simulink model "Control_Vehiculo_new_MCI_MCD"  (R2022a)
settings: Solver=FixedStepAuto  StartTime=0.0  StopTime=inf  MaxStep=0.01  RelTol=1e-3  EnableMultiTasking=on
InitFcn:
  | R=0.0875;
  | Lx=0.24;
  | Ly=0.279;
  | b=0.558;
  | r=R;
  | Ts=0.01;
  | cal_time=1;
libraries: simulink x6, simulink_need_slupdate x1, slpidlib x1, arduinolib x1
settings Model: ExtModeTrigDuration=2  Creator=eva_g  LastModifiedBy=Nuc1
settings SolverCC: AlgebraicLoopSolver=TrustRegion
settings OptimizationCC: EnhancedBackFolding=on  PassReuseOutputArgsAs=Individual arguments  ZeroExternalMemoryAtStartup=off  ZeroInternalMemoryAtStartup=off  MaxStackSize=64  OptimizeBlockOrder=speed  DifferentSizesBufferReuse=on  OptimizationCustomize=off  EfficientTunableParamExpr=on
settings DebuggingCC: ParameterTunabilityLossMsg=error  UnconnectedInputMsg=warning  UnconnectedOutputMsg=warning  UnconnectedLineMsg=warning  SFMachineParentedDataDiag=warning
settings HardwareCC: ProdBitPerInt=16  ProdBitPerPointer=16  ProdBitPerSizeT=16  ProdBitPerPtrDiffT=16  ProdLargestAtomicFloat=None  ProdWordSize=8  ProdHWDeviceType=Atmel->AVR
settings SFSimCC: MATLABDynamicMemAlloc=off
settings RTWCC: SystemTargetFile=ert.tlc  HardwareBoard=Arduino Mega 2560  TemplateMakefile=ert_default_tmf  Toolchain=Arduino AVR  BuildConfiguration=Faster Runs  DLArmComputeVersion=19.05
settings CodeAppCC: ForceParamTrailComments=on  IgnoreCustomStorageClasses=off  OperatorAnnotations=on  SimulinkDataObjDesc=on  SFDataObjDesc=on  InsertBlockDesc=on
settings ERTTargetCC: SupportContinuousTime=on  SupportVariableSizeSignals=on  ExtModeStaticAllocSize=2048

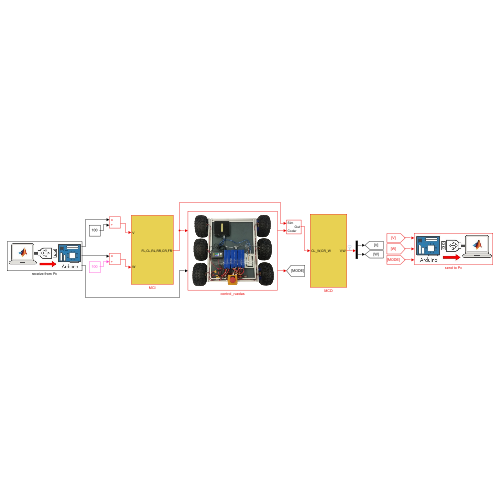
[thumbnail: Simulink's stored preview of the top-level diagram]
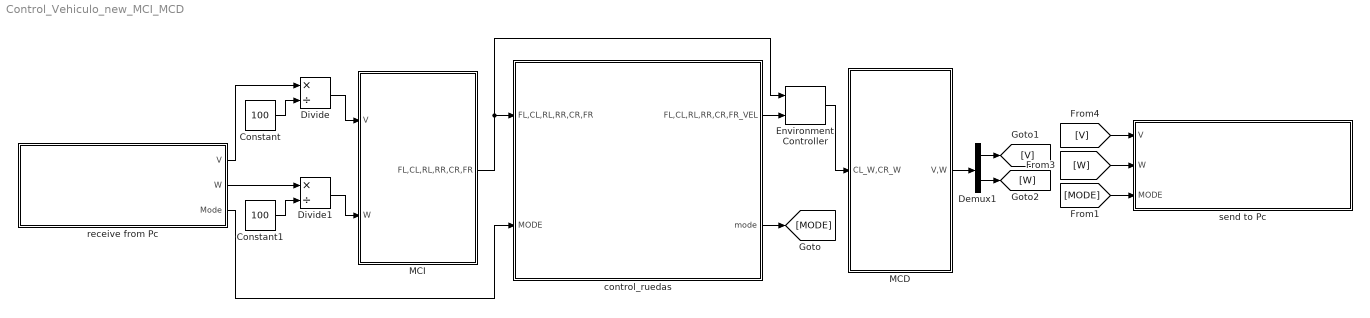
== system Control_Vehiculo_new_MCI_MCD ==
  Constant : Constant  Value=100  OutDataTypeStr=single
  Constant1 : Constant  Value=100  OutDataTypeStr=single
  Demux1 : Demux  Outputs=2
  Divide : Product  Inputs=*/
  Divide1 : Product  Inputs=*/
  Environment Controller : simulink_need_slupdate/Environment Controller
      settings: SourceProductBaseCode=SL
  MCD : Subsystem
  MCI : Subsystem
  control_ruedas : Subsystem
      mask Display: image('ruedas1.png'); % Use "Edit Image" on toolstrip to change.
  receive from Pc : Subsystem
      mask Display: image('ma.jpg'); % Use "Edit Image" on toolstrip to change.
  send to Pc : Subsystem
      mask Display: image('am.jpg'); % Use "Edit Image" on toolstrip to change.
  wires:
  [V] -> send to Pc/1(V)
  Divide1/1 -> MCI/2(W)
  Constant/1 -> Divide/2
  Divide/1 -> MCI/1(V)
  control_ruedas/1(FL,CL,RL,RR,CR,FR_VEL) -> Environment Controller/2
  MCI/1(FL,CL,RL,RR,CR,FR) -> control_ruedas/1(FL,CL,RL,RR,CR,FR), Environment Controller/1
  Environment Controller/1 -> MCD/1(CL_W,CR_W)
  Constant1/1 -> Divide1/2
  control_ruedas/2(mode) -> [MODE]
  Demux1/2 -> [W]
  [MODE] -> send to Pc/3(MODE)
  Demux1/1 -> [V]
  [W] -> send to Pc/2(W)
  MCD/1(V,W) -> Demux1/1
  receive from Pc/1(V) -> Divide/1
  receive from Pc/2(W) -> Divide1/1
  receive from Pc/3(Mode) -> control_ruedas/2(MODE)

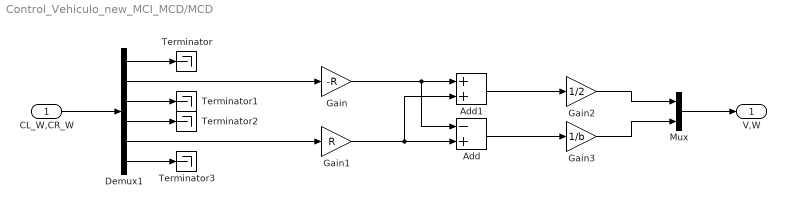
== system Control_Vehiculo_new_MCI_MCD/MCD ==
  CL_W,CR_W : Inport
  Add : Sum  Inputs=-+
  Add1 : Sum
  Demux1 : Demux  Outputs=6
  Gain : Gain  Gain=-R
  Gain1 : Gain  Gain=R
  Gain2 : Gain  Gain=1/2
  Gain3 : Gain  Gain=1/b  ParamDataTypeStr=double
  Mux : Mux  Inputs=2
  Terminator{,1..3} (4 alike) : Terminator
  V,W : Outport
  wires:
  Gain1/1 -> Add/2, Add1/2
  Gain/1 -> Add/1, Add1/1
  Add/1 -> Gain3/1
  Add1/1 -> Gain2/1
  Gain2/1 -> Mux/1
  Gain3/1 -> Mux/2
  Mux/1 -> V,W/1
  CL_W,CR_W/1 -> Demux1/1
  Demux1/2 -> Gain/1
  Demux1/5 -> Gain1/1
  Demux1/1 -> Terminator/1
  Demux1/3 -> Terminator1/1
  Demux1/4 -> Terminator2/1
  Demux1/6 -> Terminator3/1

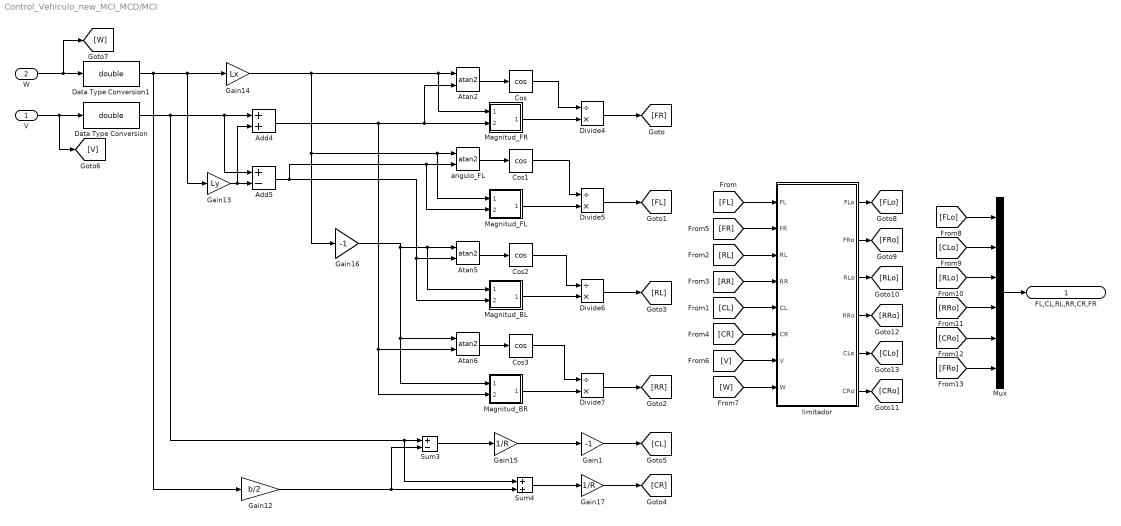
== system Control_Vehiculo_new_MCI_MCD/MCI ==
  V : Inport
  W : Inport  Port=2
  Add4 : Sum
  Add5 : Sum  Inputs=+-
  Atan2 : Trigonometry  Operator=atan2
  Atan5 : Trigonometry  Operator=atan2
  Atan6 : Trigonometry  Operator=atan2
  Cos{,1..3} (4 alike) : Trigonometry  Operator=cos
  Data Type Conversion : DataTypeConversion  OutDataTypeStr=double  SaturateOnIntegerOverflow=off  RndMeth=Floor
  Data Type Conversion1 : DataTypeConversion  OutDataTypeStr=double  SaturateOnIntegerOverflow=off  RndMeth=Floor
  Divide{4..7} (4 alike) : Product  Inputs=/*
  Gain1 : Gain  Gain=-1
  Gain12 : Gain  Gain=b/2
  Gain13 : Gain  Gain=Ly
  Gain14 : Gain  Gain=Lx
  Gain15 : Gain  Gain=1/R
  Gain16 : Gain  Gain=-1
  Gain17 : Gain  Gain=1/R
  Magnitud_BL : Subsystem
  Magnitud_BR : Subsystem
  Magnitud_FL : Subsystem
  Magnitud_FR : Subsystem
  Mux : Mux  Inputs=6
  Sum3 : Sum  Inputs=+-
  Sum4 : Sum
  angulo_FL : Trigonometry  Operator=atan2
  limitador : MATLAB Function  TreatAsAtomicUnit=on
  FL,CL,RL,RR,CR,FR : Outport
  wires:
  Cos/1 -> Divide4/1
  Sum3/1 -> Gain15/1
  Cos3/1 -> Divide7/1
  Sum4/1 -> Gain17/1
  W/1 -> [W], Data Type Conversion1/1
  Gain14/1 -> Magnitud_FR/1(In1), Atan2/1, angulo_FL/1, Magnitud_FL/1(In1), Gain16/1
  Magnitud_FL/1(w_FL) -> Divide5/2
  Atan5/1 -> Cos2/1
  Gain12/1 -> Sum4/2, Sum3/2
  Gain16/1 -> Atan5/1, Magnitud_BL/1(In1), Atan6/1, Magnitud_BR/1(In1)
  Add5/1 -> angulo_FL/2, Magnitud_FL/2(In2), Atan5/2, Magnitud_BL/2(In2)
  Gain15/1 -> Gain1/1
  Add4/1 -> Atan6/2, Magnitud_BR/2(In2), Atan2/2, Magnitud_FR/2(In2)
  angulo_FL/1 -> Cos1/1
  Magnitud_BL/1(w_BL) -> Divide6/2
  Gain13/1 -> Add4/2, Add5/2
  V/1 -> [V], Data Type Conversion/1
  Cos2/1 -> Divide6/1
  Cos1/1 -> Divide5/1
  Magnitud_BR/1(w_BR) -> Divide7/2
  Magnitud_FR/1(w_FR) -> Divide4/2
  Atan6/1 -> Cos3/1
  Atan2/1 -> Cos/1
  Mux/1 -> FL,CL,RL,RR,CR,FR/1
  Divide4/1 -> [FR]
  Divide5/1 -> [FL]
  Divide6/1 -> [RL]
  Gain1/1 -> [CL]
  Gain17/1 -> [CR]
  Data Type Conversion/1 -> Sum4/1, Sum3/1, Add5/1, Add4/1
  Data Type Conversion1/1 -> Gain12/1, Gain14/1, Gain13/1
  Divide7/1 -> [RR]
  [CR] -> limitador/6(CR)
  [FR] -> limitador/2(FR)
  [CL] -> limitador/5(CL)
  [RL] -> limitador/3(RL)
  [FL] -> limitador/1(FL)
  [RR] -> limitador/4(RR)
  [V] -> limitador/7(V)
  [W] -> limitador/8(W)
  limitador/1(FLo) -> [FLo]
  limitador/2(FRo) -> [FRo]
  limitador/3(RLo) -> [RLo]
  limitador/4(RRo) -> [RRo]
  limitador/5(CLo) -> [CLo]
  limitador/6(CRo) -> [CRo]
  [FLo] -> Mux/1
  [CLo] -> Mux/2
  [RLo] -> Mux/3
  [CRo] -> Mux/5
  [FRo] -> Mux/6
  [RRo] -> Mux/4

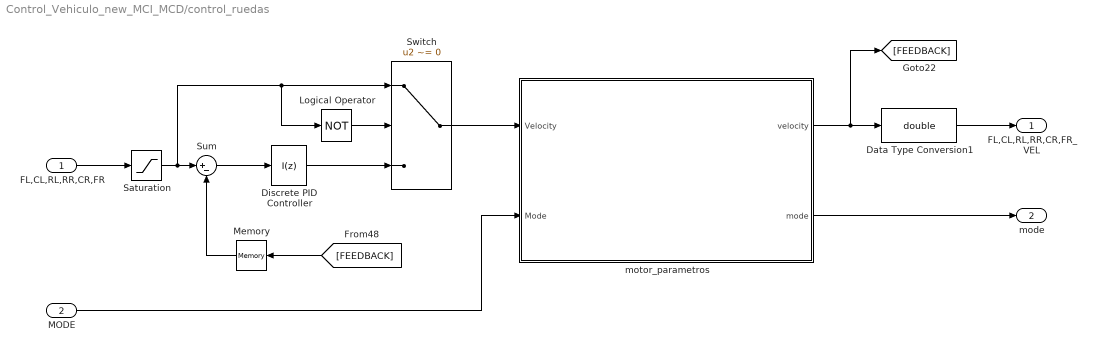
== system Control_Vehiculo_new_MCI_MCD/control_ruedas ==
  FL,CL,RL,RR,CR,FR : Inport
  MODE : Inport  Port=2
  Data Type Conversion1 : DataTypeConversion  OutDataTypeStr=double  SaturateOnIntegerOverflow=off  RndMeth=Floor
  Discrete PID Controller : slpidlib/PID Controller  Controller=I  Form=Parallel  TimeDomain=Discrete-time  UseExternalTs=off  SampleTime=-1  IntegratorMethod=Forward Euler  FilterMethod=Forward Euler  ControllerParametersSource=internal  P=0.7  I=10  UseKiTs=off  D=0  N=100  UseFilter=on  TunerSelectOption=Transfer Function Based (PID Tuner App)  InitialConditionSource=internal  InitialConditionForIntegrator=0  InitialConditionForFilter=0  DifferentiatorICPrevScaledInput=0  ExternalReset=none  TrackingMode=off  Kt=1  LimitOutput=on  SatLimitsSource=internal  UpperSaturationLimit=10  LowerSaturationLimit=-10  LinearizeAsGain=on  AntiWindupMode=clamping  Kb=1  POutMin=[]  POutMax=[]  IOutMin=[]  IOutMax=[]  DOutMin=[]  DOutMax=[]  NOutMin=[]  NOutMax=[]  SumOutMin=[]  SumOutMax=[]  SaturationOutMin=[]  SaturationOutMax=[]  PParamMin=[]  PParamMax=[]  IParamMin=[]  IParamMax=[]  DParamMin=[]  DParamMax=[]  NParamMin=[]  NParamMax=[]  KbParamMin=[]  KbParamMax=[]  KtParamMin=[]  KtParamMax=[]  KbOutMin=[]  KbOutMax=[]  KtOutMin=[]  KtOutMax=[]  IntegratorOutMin=[]  IntegratorOutMax=[]  FilterOutMin=[]  FilterOutMax=[]  SumI1OutMin=[]  SumI1OutMax=[]  SumI2OutMin=[]  SumI2OutMax=[]  SumI3OutMin=[]  SumI3OutMax=[]  SumI4OutMin=[]  SumI4OutMax=[]  SumDOutMin=[]  SumDOutMax=[]  DifferentiatorOutMin=[]  DifferentiatorOutMax=[]  FilterDiffOutCoefMin=[]  FilterDiffOutCoefMax=[]  ReciprocalOutMin=[]  ReciprocalOutMax=[]  SumDenOutMin=[]  SumDenOutMax=[]  SumNumOutMin=[]  SumNumOutMax=[]  DivideOutMin=[]  DivideOutMax=[]  UdiffTsProdOutMin=[]  UdiffTsProdOutMax=[]  NTsProdOutMin=[]  NTsProdOutMax=[]  UintegralTsProdOutMin=[]  UintegralTsProdOutMax=[]  UngainTsProdOutMin=[]  UngainTsProdOutMax=[]  IntegratorContinuousStateAttributes=''  IntegratorStateMustResolveToSignalObject=off  IntegratorRTWStateStorageClass=Auto  FilterContinuousStateAttributes=''  FilterStateMustResolveToSignalObject=off  FilterRTWStateStorageClass=Auto  ParallelPVariant=Disabled  IdealPVariant=Disabled  IVariant=InternalParameters  DVariant=Disabled  IntegratorVariant=Discrete  SatVariant=Enabled  AWVariant=DiscClampingParallel  PCopyVariant=Disabled  TRVariant=Disabled  FdbkBlocksVariant=Forward  IdealPFdbkVariant=Disabled  SatFdbkVariant=Disabled  DerivativeFilterVariant=Disabled  NVariant=Disabled  NCopyVariant=Disabled_SignalSpec  FilterICVariant=Disabled  IntegratorICVariant=InternalICs  ExternalResetVariant=Disabled  TRSumVariant=Passthrough  SumFdbkVariant=Disabled  SumVariant=Passthrough_I  TsampFilterVariant=InternalTs  TsampNgainVariant=Passthrough  TsampIntegralVariant=Passthrough  ExternalSaturationOutDataTypeStr=Inherit: Same as second input  aMode=0
  Logical Operator : Logic  Operator=NOT  AllPortsSameDT=off  OutDataTypeStr=boolean
  Memory : Memory
  Saturation : Saturate  UpperLimit=10  LowerLimit=-10
  Sum : Sum  Inputs=|+-
  Switch : Switch  Criteria=u2 ~= 0  SaturateOnIntegerOverflow=off  InputSameDT=off
  motor_parametros : Subsystem
  FL,CL,RL,RR,CR,FR_VEL : Outport
  mode : Outport  Port=2
  wires:
  Memory/1 -> Sum/2
  Sum/1 -> Discrete PID Controller/1
  Discrete PID Controller/1 -> Switch/3
  [FEEDBACK] -> Memory/1
  Data Type Conversion1/1 -> FL,CL,RL,RR,CR,FR_VEL/1
  Logical Operator/1 -> Switch/2
  FL,CL,RL,RR,CR,FR/1 -> Saturation/1
  Saturation/1 -> Logical Operator/1, Switch/1, Sum/1
  motor_parametros/1(velocity) -> [FEEDBACK], Data Type Conversion1/1
  MODE/1 -> motor_parametros/2(Mode)
  motor_parametros/2(mode) -> mode/1
  Switch/1 -> motor_parametros/1(Velocity)

== system Control_Vehiculo_new_MCI_MCD/receive from Pc ==
  receive from Pc : S-Function  InitFcn=try, set_param(gcb,'FunctionName','receive_serial'), end  FunctionName=receive_serial  SFunctionModules=receive_serial_wrapper  SFunctionDeploymentMode=off  EnableBusSupport=off  mask(S-Function Builder){}
      mask help: Simulink:masks:SFunctionBuilder_MD
      mask init:
      | val = [[.9  0.75 0.75 1 1 .9 .9 1]',[1 1 0.75 0.75 .9 .9 1 .9]'];try , sys = get_param(gcb,'SfunBuilderFcnName');if isempty(sys), sys = get_param(gcb,'FunctionName'); end,catch, sys = get_param(gcb,'FunctionName'); end
      settings: CopyFcn=set_param(gcbh,'LinkStatus','none')  PreSaveFcn=try, set_param(gcb,'FunctionName','receive_serial'), end  OpenFcn=sfunctionwizard(gcbh)
      mask Display: plot(val(:,1),val(:,2)),disp(sys),port_label('output',1,'v'),port_label('output',2,'w'),port_label('output',3,'m')
  V : Outport
  W : Outport  Port=2
  Mode : Outport  Port=3
  wires:
  receive from Pc/2 -> W/1
  receive from Pc/1 -> V/1
  receive from Pc/3 -> Mode/1

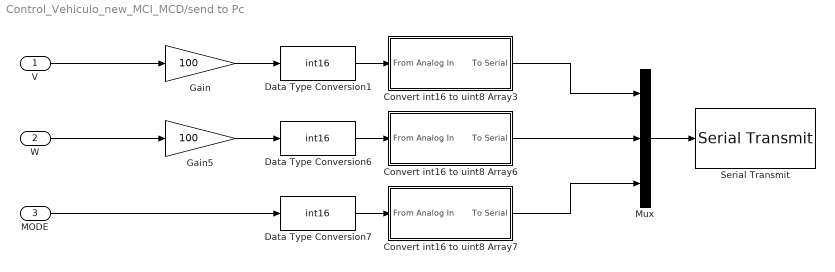
== system Control_Vehiculo_new_MCI_MCD/send to Pc ==
  V : Inport
  W : Inport  Port=2
  MODE : Inport  Port=3
  Convert int16 to uint8 Array3 : Subsystem
  Convert int16 to uint8 Array6 : Subsystem
  Convert int16 to uint8 Array7 : Subsystem
  Data Type Conversion1 : DataTypeConversion  OutDataTypeStr=int16  ConvertRealWorld=Stored Integer (SI)  SaturateOnIntegerOverflow=off  RndMeth=Floor
  Data Type Conversion6 : DataTypeConversion  OutDataTypeStr=int16  ConvertRealWorld=Stored Integer (SI)  SaturateOnIntegerOverflow=off  RndMeth=Floor
  Data Type Conversion7 : DataTypeConversion  OutDataTypeStr=int16  ConvertRealWorld=Stored Integer (SI)  SaturateOnIntegerOverflow=off  RndMeth=Floor
  Gain : Gain  Gain=100
  Gain5 : Gain  Gain=100
  Mux : Mux  Inputs=3
  Serial Transmit : arduinolib/Serial Transmit  portNumber=0  sendmode=write  sendformat=Decimal  floatprecision=2  blockPlatform=arduino
  wires:
  Convert int16 to uint8 Array7/1(To Serial) -> Mux/3
  Data Type Conversion7/1 -> Convert int16 to uint8 Array7/1(From Analog In)
  MODE/1 -> Data Type Conversion7/1
  W/1 -> Gain5/1
  V/1 -> Gain/1
  Convert int16 to uint8 Array3/1(To Serial) -> Mux/1
  Convert int16 to uint8 Array6/1(To Serial) -> Mux/2
  Gain5/1 -> Data Type Conversion6/1
  Data Type Conversion6/1 -> Convert int16 to uint8 Array6/1(From Analog In)
  Gain/1 -> Data Type Conversion1/1
  Data Type Conversion1/1 -> Convert int16 to uint8 Array3/1(From Analog In)
  Mux/1 -> Serial Transmit/1

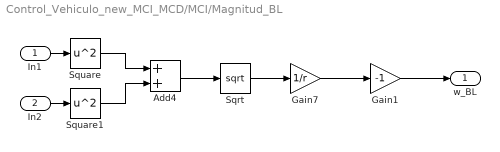
== system Control_Vehiculo_new_MCI_MCD/MCI/Magnitud_BL ==
  In1 : Inport
  In2 : Inport  Port=2
  Add4 : Sum
  Gain1 : Gain  Gain=-1
  Gain7 : Gain  Gain=1/r
  Sqrt : Sqrt
  Square : Math  Operator=square
  Square1 : Math  Operator=square
  w_BL : Outport
  wires:
  Sqrt/1 -> Gain7/1
  Square1/1 -> Add4/2
  In2/1 -> Square1/1
  Add4/1 -> Sqrt/1
  Square/1 -> Add4/1
  In1/1 -> Square/1
  Gain7/1 -> Gain1/1
  Gain1/1 -> w_BL/1

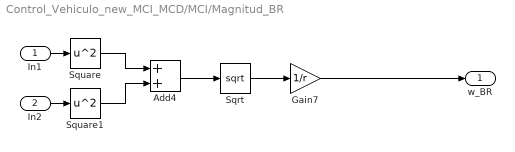
== system Control_Vehiculo_new_MCI_MCD/MCI/Magnitud_BR ==
  In1 : Inport
  In2 : Inport  Port=2
  Add4 : Sum
  Gain7 : Gain  Gain=1/r
  Sqrt : Sqrt
  Square : Math  Operator=square
  Square1 : Math  Operator=square
  w_BR : Outport
  wires:
  In1/1 -> Square/1
  Square/1 -> Add4/1
  Add4/1 -> Sqrt/1
  In2/1 -> Square1/1
  Square1/1 -> Add4/2
  Sqrt/1 -> Gain7/1
  Gain7/1 -> w_BR/1

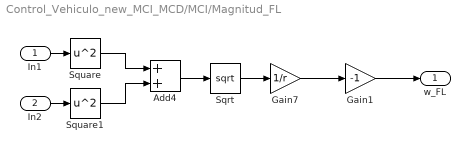
== system Control_Vehiculo_new_MCI_MCD/MCI/Magnitud_FL ==
  In1 : Inport
  In2 : Inport  Port=2
  Add4 : Sum
  Gain1 : Gain  Gain=-1
  Gain7 : Gain  Gain=1/r
  Sqrt : Sqrt
  Square : Math  Operator=square
  Square1 : Math  Operator=square
  w_FL : Outport
  wires:
  Square1/1 -> Add4/2
  In2/1 -> Square1/1
  Add4/1 -> Sqrt/1
  Square/1 -> Add4/1
  In1/1 -> Square/1
  Sqrt/1 -> Gain7/1
  Gain7/1 -> Gain1/1
  Gain1/1 -> w_FL/1

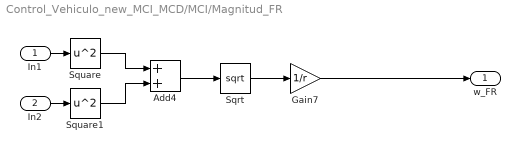
== system Control_Vehiculo_new_MCI_MCD/MCI/Magnitud_FR ==
  In1 : Inport
  In2 : Inport  Port=2
  Add4 : Sum
  Gain7 : Gain  Gain=1/r
  Sqrt : Sqrt
  Square : Math  Operator=square
  Square1 : Math  Operator=square
  w_FR : Outport
  wires:
  In1/1 -> Square/1
  Square/1 -> Add4/1
  Add4/1 -> Sqrt/1
  In2/1 -> Square1/1
  Square1/1 -> Add4/2
  Sqrt/1 -> Gain7/1
  Gain7/1 -> w_FR/1

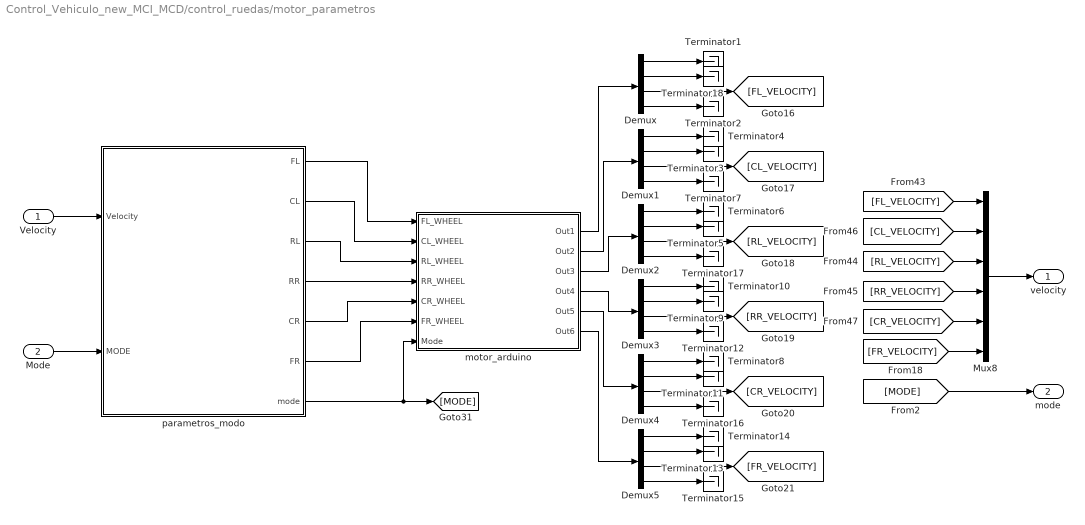
== system Control_Vehiculo_new_MCI_MCD/control_ruedas/motor_parametros ==
  Velocity : Inport
  Mode : Inport  Port=2
  Demux{,1..5} (6 alike) : Demux
  Mux8 : Mux  Inputs=6
  Terminator{1..18} (18 alike) : Terminator
  motor_arduino : Subsystem
      mask Display: image('motor.jpg'); % Use "Edit Image" on toolstrip to change.
  parametros_modo : Subsystem
  velocity : Outport
  mode : Outport  Port=2
  wires:
  [CL_VELOCITY] -> Mux8/2
  [FR_VELOCITY] -> Mux8/6
  Demux4/1 -> Terminator8/1
  parametros_modo/6(FR) -> motor_arduino/6(FR_WHEEL)
  [RL_VELOCITY] -> Mux8/3
  Demux/1 -> Terminator1/1
  parametros_modo/2(CL) -> motor_arduino/2(CL_WHEEL)
  parametros_modo/5(CR) -> motor_arduino/5(CR_WHEEL)
  Demux1/3 -> [CL_VELOCITY]
  motor_arduino/5(Out5) -> Demux4/1
  parametros_modo/1(FL) -> motor_arduino/1(FL_WHEEL)
  motor_arduino/3(Out3) -> Demux2/1
  [RR_VELOCITY] -> Mux8/4
  parametros_modo/4(RR) -> motor_arduino/4(RR_WHEEL)
  Demux2/3 -> [RL_VELOCITY]
  Demux1/2 -> Terminator3/1
  motor_arduino/1(Out1) -> Demux/1
  parametros_modo/3(RL) -> motor_arduino/3(RL_WHEEL)
  Demux3/2 -> Terminator9/1
  Demux/2 -> Terminator18/1
  [CR_VELOCITY] -> Mux8/5
  [FL_VELOCITY] -> Mux8/1
  Demux2/2 -> Terminator5/1
  Demux/3 -> [FL_VELOCITY]
  Demux3/3 -> [RR_VELOCITY]
  Demux1/1 -> Terminator4/1
  Demux3/1 -> Terminator10/1
  Demux/4 -> Terminator2/1
  motor_arduino/2(Out2) -> Demux1/1
  Demux4/3 -> [CR_VELOCITY]
  Demux5/2 -> Terminator13/1
  motor_arduino/4(Out4) -> Demux3/1
  Demux3/4 -> Terminator12/1
  Demux2/1 -> Terminator6/1
  motor_arduino/6(Out6) -> Demux5/1
  Demux5/3 -> [FR_VELOCITY]
  Demux5/4 -> Terminator15/1
  Demux5/1 -> Terminator14/1
  Demux4/4 -> Terminator16/1
  Demux4/2 -> Terminator11/1
  Demux2/4 -> Terminator17/1
  Demux1/4 -> Terminator7/1
  Mux8/1 -> velocity/1
  Velocity/1 -> parametros_modo/1(Velocity)
  Mode/1 -> parametros_modo/2(MODE)
  parametros_modo/7(mode) -> [MODE], motor_arduino/7(Mode)
  [MODE] -> mode/1

== system Control_Vehiculo_new_MCI_MCD/send to Pc/Convert int16 to uint8 Array3 ==
  From Analog In : Inport
  Data Type Conversion1 : DataTypeConversion  OutDataTypeStr=uint8  ConvertRealWorld=Stored Integer (SI)  SaturateOnIntegerOverflow=off  RndMeth=Floor
  Data Type Conversion2 : DataTypeConversion  OutDataTypeStr=uint8  ConvertRealWorld=Stored Integer (SI)  SaturateOnIntegerOverflow=off  RndMeth=Floor
  Extract Bits : simulink/Logic and Bit Operations/Extract Bits  bitsToExtract=Upper half  numBits=8  bitIdxRange=[0 7]  outScalingMode=Treat bit field as an integer
  Extract Bits1 : simulink/Logic and Bit Operations/Extract Bits  bitsToExtract=Lower half  numBits=8  bitIdxRange=[0 7]  outScalingMode=Treat bit field as an integer
  Mux : Mux  Inputs=2
  To Serial : Outport
  wires:
  From Analog In/1 -> Extract Bits/1, Extract Bits1/1
  Extract Bits1/1 -> Data Type Conversion1/1
  Extract Bits/1 -> Data Type Conversion2/1
  Data Type Conversion1/1 -> Mux/1
  Data Type Conversion2/1 -> Mux/2
  Mux/1 -> To Serial/1

== system Control_Vehiculo_new_MCI_MCD/send to Pc/Convert int16 to uint8 Array6 ==
  From Analog In : Inport
  Data Type Conversion1 : DataTypeConversion  OutDataTypeStr=uint8  ConvertRealWorld=Stored Integer (SI)  SaturateOnIntegerOverflow=off  RndMeth=Floor
  Data Type Conversion2 : DataTypeConversion  OutDataTypeStr=uint8  ConvertRealWorld=Stored Integer (SI)  SaturateOnIntegerOverflow=off  RndMeth=Floor
  Extract Bits : simulink/Logic and Bit Operations/Extract Bits  bitsToExtract=Upper half  numBits=8  bitIdxRange=[0 7]  outScalingMode=Treat bit field as an integer
  Extract Bits1 : simulink/Logic and Bit Operations/Extract Bits  bitsToExtract=Lower half  numBits=8  bitIdxRange=[0 7]  outScalingMode=Treat bit field as an integer
  Mux : Mux  Inputs=2
  To Serial : Outport
  wires:
  From Analog In/1 -> Extract Bits/1, Extract Bits1/1
  Extract Bits1/1 -> Data Type Conversion1/1
  Extract Bits/1 -> Data Type Conversion2/1
  Data Type Conversion1/1 -> Mux/1
  Data Type Conversion2/1 -> Mux/2
  Mux/1 -> To Serial/1

== system Control_Vehiculo_new_MCI_MCD/send to Pc/Convert int16 to uint8 Array7 ==
  From Analog In : Inport
  Data Type Conversion1 : DataTypeConversion  OutDataTypeStr=uint8  ConvertRealWorld=Stored Integer (SI)  SaturateOnIntegerOverflow=off  RndMeth=Floor
  Data Type Conversion2 : DataTypeConversion  OutDataTypeStr=uint8  ConvertRealWorld=Stored Integer (SI)  SaturateOnIntegerOverflow=off  RndMeth=Floor
  Extract Bits : simulink/Logic and Bit Operations/Extract Bits  bitsToExtract=Upper half  numBits=8  bitIdxRange=[0 7]  outScalingMode=Treat bit field as an integer
  Extract Bits1 : simulink/Logic and Bit Operations/Extract Bits  bitsToExtract=Lower half  numBits=8  bitIdxRange=[0 7]  outScalingMode=Treat bit field as an integer
  Mux : Mux  Inputs=2
  To Serial : Outport
  wires:
  From Analog In/1 -> Extract Bits/1, Extract Bits1/1
  Extract Bits1/1 -> Data Type Conversion1/1
  Extract Bits/1 -> Data Type Conversion2/1
  Data Type Conversion1/1 -> Mux/1
  Data Type Conversion2/1 -> Mux/2
  Mux/1 -> To Serial/1

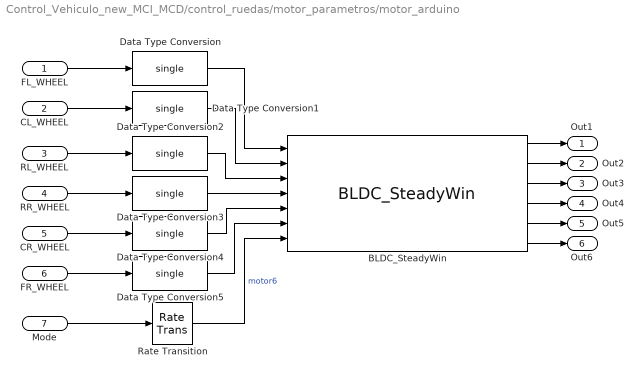
== system Control_Vehiculo_new_MCI_MCD/control_ruedas/motor_parametros/motor_arduino ==
  FL_WHEEL : Inport
  CL_WHEEL : Inport  Port=2
  RL_WHEEL : Inport  Port=3
  RR_WHEEL : Inport  Port=4
  CR_WHEEL : Inport  Port=5
  FR_WHEEL : Inport  Port=6
  Mode : Inport  Port=7
  BLDC_SteadyWin : S-Function  InitFcn=try, set_param(gcb,'FunctionName','BLDC_SteadyWin'), end  FunctionName=BLDC_SteadyWin  SFunctionModules=BLDC_SteadyWin_wrapper  SFunctionDeploymentMode=off  EnableBusSupport=off  mask(S-Function Builder){}
      mask help: Simulink:masks:SFunctionBuilder_MD
      mask init: same as Control_Vehiculo_new_MCI_MCD/receive from Pc/receive from Pc
      settings: CopyFcn=set_param(gcbh,'LinkStatus','none')  PreSaveFcn=try, set_param(gcb,'FunctionName','BLDC_SteadyWin'), end  OpenFcn=sfunctionwizard(gcbh)
      mask Display:
      | plot(val(:,1),val(:,2))
      | disp(sys)
      | port_label('input',1,'In1')
      | port_label('input',2,'In2')
      | port_label('input',3,'In3')
      | port_label('input',4,'In4')
      | port_label('input',5,'In5')
      | port_label('input',6,'In6')
      | port_label('input',7,'Mode')
      | port_label('output',1,'Out1')
      | port_label('output',2,'Out2')
      | port_label('output',3,'Out3')
      | port_label('output',4,'Out4')
      | port_label('output',5,'Out5')
      | port_label('output',6,'Out6')
  Data Type Conversion{,1..5} (6 alike) : DataTypeConversion  OutDataTypeStr=single  SaturateOnIntegerOverflow=off  RndMeth=Floor
  Rate Transition : RateTransition
  Out1 : Outport
  Out2 : Outport  Port=2
  Out3 : Outport  Port=3
  Out4 : Outport  Port=4
  Out5 : Outport  Port=5
  Out6 : Outport  Port=6
  wires:
  FL_WHEEL/1 -> Data Type Conversion/1
  BLDC_SteadyWin/1 -> Out1/1
  BLDC_SteadyWin/2 -> Out2/1
  BLDC_SteadyWin/3 -> Out3/1
  BLDC_SteadyWin/4 -> Out4/1
  BLDC_SteadyWin/5 -> Out5/1
  BLDC_SteadyWin/6 -> Out6/1
  CL_WHEEL/1 -> Data Type Conversion1/1
  Data Type Conversion1/1 -> BLDC_SteadyWin/2
  Data Type Conversion/1 -> BLDC_SteadyWin/1
  Mode/1 -> Rate Transition/1
  Data Type Conversion3/1 -> BLDC_SteadyWin/4
  Data Type Conversion2/1 -> BLDC_SteadyWin/3
  RL_WHEEL/1 -> Data Type Conversion2/1
  RR_WHEEL/1 -> Data Type Conversion3/1
  Data Type Conversion5/1 -> BLDC_SteadyWin/6
  Data Type Conversion4/1 -> BLDC_SteadyWin/5
  CR_WHEEL/1 -> Data Type Conversion4/1
  FR_WHEEL/1 -> Data Type Conversion5/1
  Rate Transition/1 -> BLDC_SteadyWin/7  "motor6"

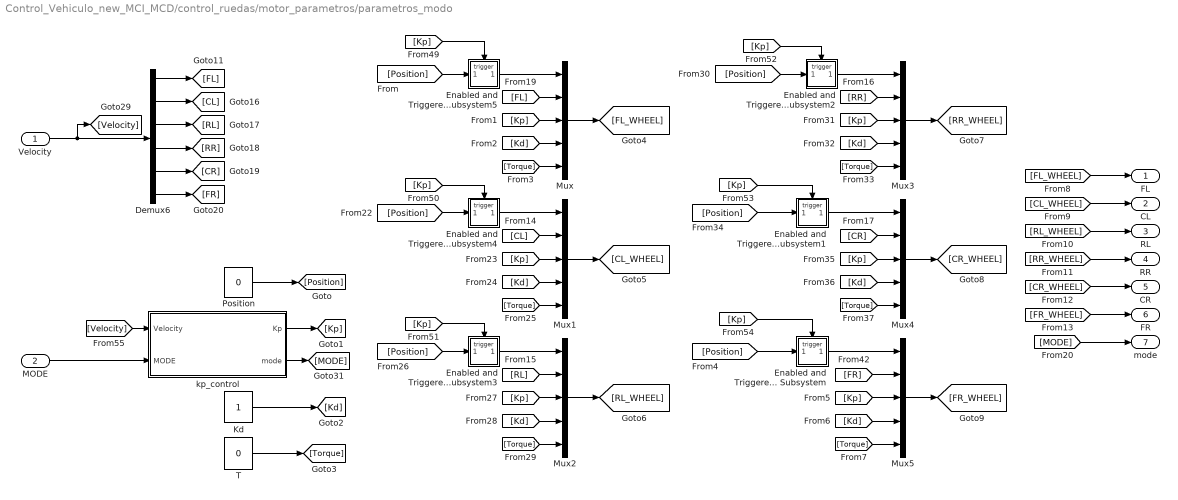
== system Control_Vehiculo_new_MCI_MCD/control_ruedas/motor_parametros/parametros_modo ==
  Velocity : Inport
  MODE : Inport  Port=2
  Demux6 : Demux  Outputs=6
  Enabled and Triggered Subsystem : Subsystem  TreatAsAtomicUnit=on
  Enabled and Triggered Subsystem1 : Subsystem  TreatAsAtomicUnit=on
  Enabled and Triggered Subsystem2 : Subsystem  TreatAsAtomicUnit=on
  Enabled and Triggered Subsystem3 : Subsystem  TreatAsAtomicUnit=on
  Enabled and Triggered Subsystem4 : Subsystem  TreatAsAtomicUnit=on
  Enabled and Triggered Subsystem5 : Subsystem  TreatAsAtomicUnit=on
  Kd : Constant  SampleTime=-1
  Mux{,1..5} (6 alike) : Mux  Inputs=5
  Position : Constant  Value=0  SampleTime=-1
  T : Constant  Value=0  SampleTime=-1
  kp_control : Subsystem
  FL : Outport
  CL : Outport  Port=2
  RL : Outport  Port=3
  RR : Outport  Port=4
  CR : Outport  Port=5
  FR : Outport  Port=6
  mode : Outport  Port=7
  wires:
  [Kp] -> Mux/3
  [RR] -> Mux3/2
  [Kp] -> Mux3/3
  [Torque] -> Mux3/5
  [Torque] -> Mux4/5
  [RL] -> Mux2/2
  Enabled and Triggered Subsystem3/1(Out1) -> Mux2/1
  [Kd] -> Mux2/4
  Mux1/1 -> [CL_WHEEL]
  [Kp] -> Mux4/3
  [Torque] -> Mux1/5
  [Kd] -> Mux1/4
  Mux5/1 -> [FR_WHEEL]
  [Kp] -> Mux1/3
  Mux2/1 -> [RL_WHEEL]
  [CR] -> Mux4/2
  [Torque] -> Mux2/5
  [FL] -> Mux/2
  [Kd] -> Mux/4
  Mux4/1 -> [CR_WHEEL]
  [Position] -> Enabled and Triggered Subsystem1/1(In1)
  [Kd] -> Mux4/4
  [Kp] -> Mux2/3
  [Torque] -> Mux/5
  Enabled and Triggered Subsystem4/1(Out1) -> Mux1/1
  Enabled and Triggered Subsystem/1(Out1) -> Mux5/1
  Mux3/1 -> [RR_WHEEL]
  Enabled and Triggered Subsystem5/1(Out1) -> Mux/1
  [Kd] -> Mux3/4
  [CL] -> Mux1/2
  [Kd] -> Mux5/4
  [Position] -> Enabled and Triggered Subsystem5/1(In1)
  [Position] -> Enabled and Triggered Subsystem/1(In1)
  [Kp] -> Enabled and Triggered Subsystem1/Trigger
  [FR] -> Mux5/2
  [Kp] -> Enabled and Triggered Subsystem4/Trigger
  Enabled and Triggered Subsystem1/1(Out1) -> Mux4/1
  [Position] -> Enabled and Triggered Subsystem2/1(In1)
  [Torque] -> Mux5/5
  [Kp] -> Enabled and Triggered Subsystem3/Trigger
  [Position] -> Enabled and Triggered Subsystem4/1(In1)
  [Kp] -> Mux5/3
  [Position] -> Enabled and Triggered Subsystem3/1(In1)
  Mux/1 -> [FL_WHEEL]
  [Kp] -> Enabled and Triggered Subsystem5/Trigger
  [Kp] -> Enabled and Triggered Subsystem/Trigger
  Enabled and Triggered Subsystem2/1(Out1) -> Mux3/1
  [Kp] -> Enabled and Triggered Subsystem2/Trigger
  Demux6/6 -> [FR]
  Demux6/1 -> [FL]
  kp_control/2(mode) -> [MODE]
  MODE/1 -> kp_control/2(MODE)
  Kd/1 -> [Kd]
  T/1 -> [Torque]
  Position/1 -> [Position]
  kp_control/1(Kp) -> [Kp]
  [Velocity] -> kp_control/1(Velocity)
  Velocity/1 -> Demux6/1, [Velocity]
  [FL_WHEEL] -> FL/1
  [CL_WHEEL] -> CL/1
  [RL_WHEEL] -> RL/1
  [RR_WHEEL] -> RR/1
  [CR_WHEEL] -> CR/1
  [FR_WHEEL] -> FR/1
  [MODE] -> mode/1
  Demux6/2 -> [CL]
  Demux6/3 -> [RL]
  Demux6/4 -> [RR]
  Demux6/5 -> [CR]

== system Control_Vehiculo_new_MCI_MCD/control_ruedas/motor_parametros/parametros_modo/Enabled and Triggered Subsystem ==
  In1 : Inport
  Trigger : TriggerPort  VariantControl=Variant
  Out1 : Outport
  wires:
  In1/1 -> Out1/1

== system Control_Vehiculo_new_MCI_MCD/control_ruedas/motor_parametros/parametros_modo/Enabled and Triggered Subsystem1 ==
  In1 : Inport
  Trigger : TriggerPort  VariantControl=Variant
  Out1 : Outport
  wires:
  In1/1 -> Out1/1

== system Control_Vehiculo_new_MCI_MCD/control_ruedas/motor_parametros/parametros_modo/Enabled and Triggered Subsystem2 ==
  In1 : Inport
  Trigger : TriggerPort  VariantControl=Variant
  Out1 : Outport
  wires:
  In1/1 -> Out1/1

== system Control_Vehiculo_new_MCI_MCD/control_ruedas/motor_parametros/parametros_modo/Enabled and Triggered Subsystem3 ==
  In1 : Inport
  Trigger : TriggerPort  VariantControl=Variant
  Out1 : Outport
  wires:
  In1/1 -> Out1/1

== system Control_Vehiculo_new_MCI_MCD/control_ruedas/motor_parametros/parametros_modo/Enabled and Triggered Subsystem4 ==
  In1 : Inport
  Trigger : TriggerPort  VariantControl=Variant
  Out1 : Outport
  wires:
  In1/1 -> Out1/1

== system Control_Vehiculo_new_MCI_MCD/control_ruedas/motor_parametros/parametros_modo/Enabled and Triggered Subsystem5 ==
  In1 : Inport
  Trigger : TriggerPort  VariantControl=Variant
  Out1 : Outport
  wires:
  In1/1 -> Out1/1

== system Control_Vehiculo_new_MCI_MCD/control_ruedas/motor_parametros/parametros_modo/kp_control ==
  Velocity : Inport
  MODE : Inport  Port=2
  Data Type Conversion1 : DataTypeConversion  OutDataTypeStr=uint8  SaturateOnIntegerOverflow=off  RndMeth=Floor
  Data Type Conversion5 : DataTypeConversion  OutDataTypeStr=double  SaturateOnIntegerOverflow=off  RndMeth=Floor
  Demux7 : Demux  Outputs=6
  Kp_control : MATLAB Function  TreatAsAtomicUnit=on
  Kp : Outport
  mode : Outport  Port=2
  wires:
  Demux7/5 -> Kp_control/5(CR)
  Demux7/6 -> Kp_control/6(FR)
  Demux7/1 -> Kp_control/1(FL)
  Demux7/2 -> Kp_control/2(CL)
  Kp_control/1(Kp) -> Kp/1
  Demux7/3 -> Kp_control/3(RL)
  Demux7/4 -> Kp_control/4(RR)
  Velocity/1 -> Demux7/1
  Kp_control/2(mode) -> Data Type Conversion1/1
  Data Type Conversion1/1 -> mode/1
  MODE/1 -> Data Type Conversion5/1
  Data Type Conversion5/1 -> Kp_control/7(MODE)

== matlab function Control_Vehiculo_new_MCI_MCD/control_ruedas/motor_parametros/parametros_modo/kp_control/Kp_control ==
  data: FL input; Kp output; CL input; RL input; RR input; CR input; FR input; MODE input size=1; mode output
function [Kp, mode] = fcn(FL,CL,RL,RR,CR,FR,MODE)

    if(FL==0) && (CL==0) && (RL==0) && (RR==0) && (CR==0) && (FR==0) && (MODE==1)
        Kp = 25;
        mode = 2;
    else
        Kp = 0;
        mode = MODE;
    end

== matlab function Control_Vehiculo_new_MCI_MCD/MCI/limitador ==
  data: FL input; FLo output; FR input; RL input; RR input; CL input; CR input; V input; W input; FRo output; RLo output; RRo output; CLo output; CRo output
function [FLo,FRo,RLo,RRo,CLo,CRo] = limitador(FL,FR,RL,RR,CL,CR,V,W)

double CLi;
double CRi;

if((V~=0) && (W~=0))
    
        CLi=CL;
        CRi=CR;
        
        if((V>0) && (CRi<0) || (V<0) && (CRi>0)) 
           CRi=0; 
        elseif((V>0) && (CLi>0) ||(V<0) && (CLi<0)) 
           CLi=0;
        end
        
        CLo=CLi;
        CRo=CRi;
        FLo=CLi;
        RLo=CLi;
        FRo=CRi;
        RRo=CRi;         
    
else
    
        FLo=FL;
        RLo=RL;
        FRo=FR;
        RRo=RR;
        CLo=CL;
        CRo=CR;
    

end
